simulink model "feedback_zd"  (R2022b)
settings: Solver=FixedStepAuto  StartTime=0.0  StopTime=15  FixedStep=0.001  RelTol=10-6
model workspace (MAT data in the model file):
  kd1 = Simulink.Parameter
  kd1.Value = 2
  kd1.DataType = 'auto'
  kd1.Complexity = 'real'
  kd1.Dimensions = [1 1]
  kd2 = Simulink.Parameter
  kd2.Value = 2
  kd2.DataType = 'auto'
  kd2.Complexity = 'real'
  kd2.Dimensions = [1 1]
  kp1 = Simulink.Parameter
  kp1.Value = 2
  kp1.DataType = 'auto'
  kp1.Complexity = 'real'
  kp1.Dimensions = [1 1]
  kp2 = Simulink.Parameter
  kp2.Value = 2
  kp2.DataType = 'auto'
  kp2.Complexity = 'real'
  kp2.Dimensions = [1 1]
values from neighbouring files (symbols this model uses):
  k_d1 = 50    [gains.m]
  k_d2 = 50    [gains.m]
  k_p1 = 30    [gains.m]
  k_p2 = 30    [gains.m]
undefined symbols (not defined in the file or in its folder): obstacle_x, obstacle_y, overtake_data, overtake_time
libraries: robotmobilelib x4
settings Model: Creator=thoma  LastModifiedBy=thoma
settings DebuggingCC: AlgebraicLoopMsg=none  UnderSpecifiedDimensionMsg=warning

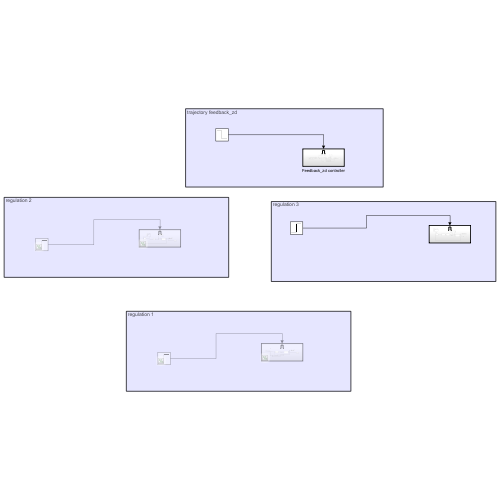
[thumbnail: Simulink's stored preview of the top-level diagram]
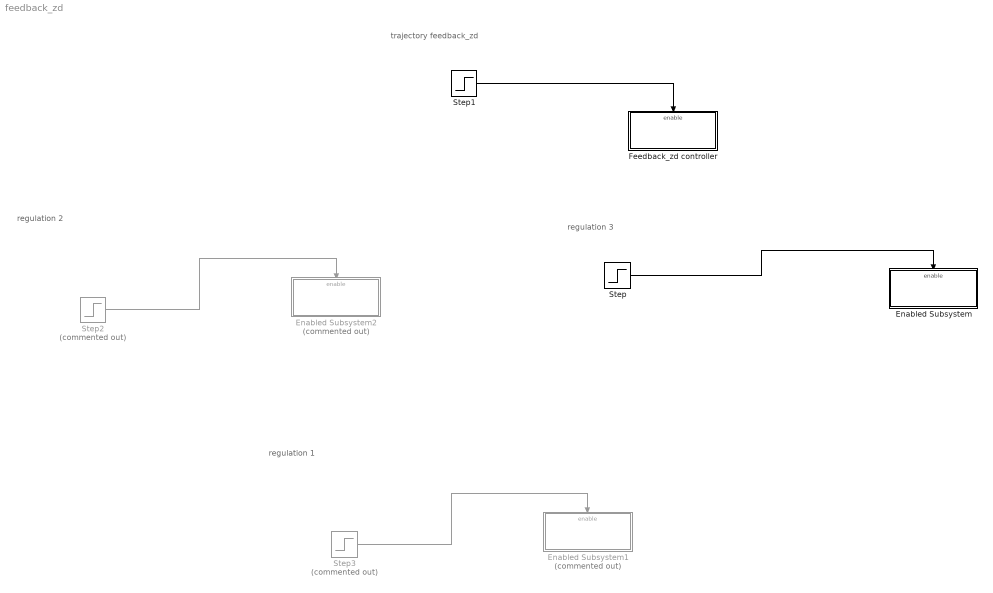
== system feedback_zd ==
  note: regulation 1
  note: regulation 3
  note: regulation 2
  note: trajectory feedback_zd
  Enabled Subsystem : Subsystem  TreatAsAtomicUnit=on
  Enabled Subsystem1 : Subsystem  Commented=on  TreatAsAtomicUnit=on
  Enabled Subsystem2 : Subsystem  Commented=on  TreatAsAtomicUnit=on
  Feedback_zd controller : Subsystem  TreatAsAtomicUnit=on
  Step : Step  Time=10  SampleTime=0
  Step1 : Step  Time=10  Before=1  After=0  SampleTime=0
  Step2 : Step  Commented=on  Time=10  SampleTime=0
  Step3 : Step  Commented=on  Time=10  SampleTime=0
  wires:
  Step3/1 -> Enabled Subsystem1/Enable
  Step1/1 -> Feedback_zd controller/Enable
  Step2/1 -> Enabled Subsystem2/Enable
  Step/1 -> Enabled Subsystem/Enable

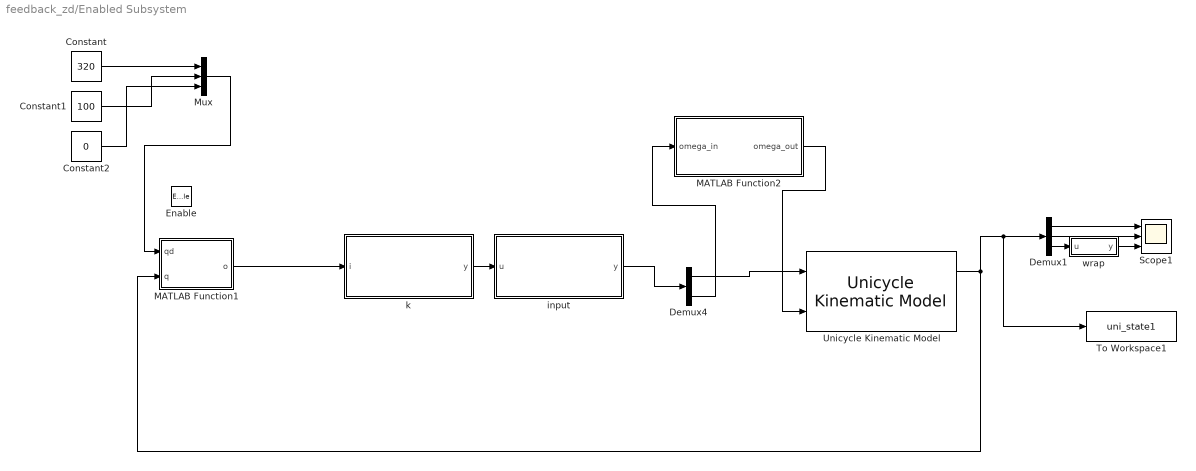
== system feedback_zd/Enabled Subsystem ==
  Enable : EnablePort
  Constant : Constant  Value=320
  Constant1 : Constant  Value=100
  Constant2 : Constant  Value=0
  Demux1 : Demux  Outputs=3
  Demux4 : Demux  Outputs=2
  MATLAB Function1 : MATLAB Function  TreatAsAtomicUnit=on
  MATLAB Function2 : MATLAB Function  TreatAsAtomicUnit=on
  Mux : Mux  Inputs=3
  Scope1 : Scope  NumInputPorts=3
  To Workspace1 : ToWorkspace  VariableName=uni_state1  SaveFormat=Structure With Time  SampleTime=0.001
  Unicycle Kinematic Model : robotmobilelib/Unicycle Kinematic Model  VehicleInputs=Vehicle Speed & Heading Angular Velocity  WheelRadius=2  WheelSpeedRange=[-Inf Inf]  InitialState=[125,60,0]  SimulateUsing=Interpreted execution
  input : MATLAB Function  TreatAsAtomicUnit=on
  k : MATLAB Function  TreatAsAtomicUnit=on
  wrap : MATLAB Function  TreatAsAtomicUnit=on
  wires:
  Constant/1 -> Mux/1
  Constant1/1 -> Mux/2
  Constant2/1 -> Mux/3
  Demux1/2 -> Scope1/2
  wrap/1(y) -> Scope1/3
  Unicycle Kinematic Model/1 -> To Workspace1/1, Demux1/1, MATLAB Function1/2(q)
  input/1(y) -> Demux4/1
  Demux1/3 -> wrap/1(u)
  k/1(y) -> input/1(u)
  Demux1/1 -> Scope1/1
  MATLAB Function1/1(o) -> k/1(i)
  Demux4/1 -> Unicycle Kinematic Model/1
  Mux/1 -> MATLAB Function1/1(qd)
  Demux4/2 -> MATLAB Function2/1(omega_in)
  MATLAB Function2/1(omega_out) -> Unicycle Kinematic Model/2

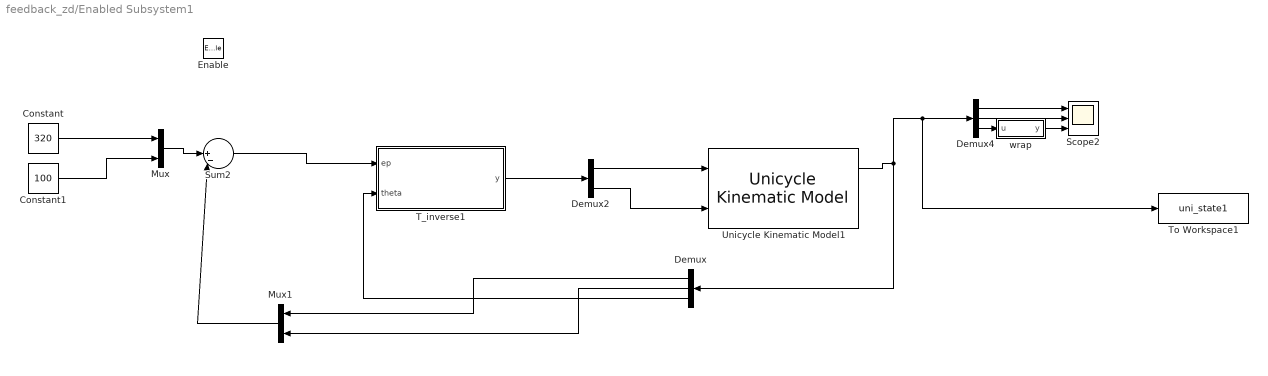
== system feedback_zd/Enabled Subsystem1 ==
  Enable : EnablePort
  Constant : Constant  Value=320
  Constant1 : Constant  Value=100
  Demux : Demux  Outputs=3
  Demux2 : Demux  Outputs=2
  Demux4 : Demux  Outputs=3
  Mux : Mux  Inputs=2
  Mux1 : Mux  Inputs=2
  Scope2 : Scope  NumInputPorts=3
  Sum2 : Sum  Inputs=||+-|
  T_inverse1 : MATLAB Function  TreatAsAtomicUnit=on
  To Workspace1 : ToWorkspace  VariableName=uni_state1  SaveFormat=Structure With Time  SampleTime=0.001
  Unicycle Kinematic Model1 : robotmobilelib/Unicycle Kinematic Model  VehicleInputs=Vehicle Speed & Heading Angular Velocity  WheelRadius=2  WheelSpeedRange=[-Inf Inf]  InitialState=[125,60,0]  SimulateUsing=Interpreted execution
  wrap : MATLAB Function  TreatAsAtomicUnit=on
  wires:
  wrap/1(y) -> Scope2/3
  Demux4/1 -> Scope2/1
  Demux4/2 -> Scope2/2
  Demux4/3 -> wrap/1(u)
  Sum2/1 -> T_inverse1/1(ep)
  Demux/1 -> Mux1/1
  Demux2/2 -> Unicycle Kinematic Model1/2
  Mux1/1 -> Sum2/2
  Demux2/1 -> Unicycle Kinematic Model1/1
  Unicycle Kinematic Model1/1 -> To Workspace1/1, Demux4/1, Demux/1
  T_inverse1/1(y) -> Demux2/1
  Demux/2 -> Mux1/2
  Demux/3 -> T_inverse1/2(theta)
  Constant1/1 -> Mux/2
  Constant/1 -> Mux/1
  Mux/1 -> Sum2/1

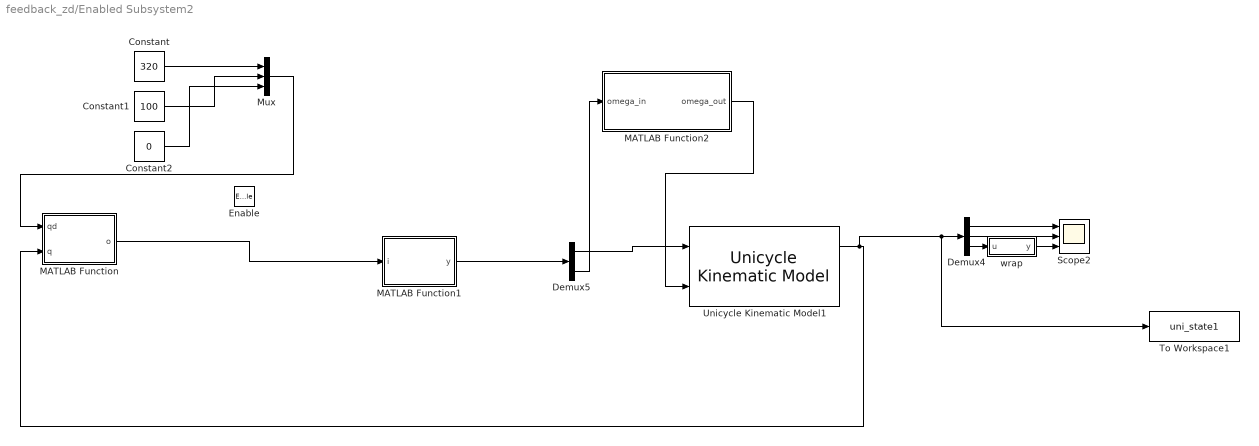
== system feedback_zd/Enabled Subsystem2 ==
  Enable : EnablePort
  Constant : Constant  Value=320
  Constant1 : Constant  Value=100
  Constant2 : Constant  Value=0
  Demux4 : Demux  Outputs=3
  Demux5 : Demux  Outputs=2
  MATLAB Function : MATLAB Function  TreatAsAtomicUnit=on
  MATLAB Function1 : MATLAB Function  TreatAsAtomicUnit=on
  MATLAB Function2 : MATLAB Function  TreatAsAtomicUnit=on
  Mux : Mux  Inputs=3
  Scope2 : Scope  NumInputPorts=3
  To Workspace1 : ToWorkspace  VariableName=uni_state1  SaveFormat=Structure With Time  SampleTime=0.001
  Unicycle Kinematic Model1 : robotmobilelib/Unicycle Kinematic Model  VehicleInputs=Vehicle Speed & Heading Angular Velocity  WheelRadius=2  WheelSpeedRange=[-Inf Inf]  InitialState=[125,60,0]  SimulateUsing=Interpreted execution
  wrap : MATLAB Function  TreatAsAtomicUnit=on
  wires:
  Demux5/1 -> Unicycle Kinematic Model1/1
  wrap/1(y) -> Scope2/3
  MATLAB Function/1(o) -> MATLAB Function1/1(i)
  MATLAB Function1/1(y) -> Demux5/1
  Demux4/1 -> Scope2/1
  Demux4/2 -> Scope2/2
  Demux4/3 -> wrap/1(u)
  Unicycle Kinematic Model1/1 -> To Workspace1/1, Demux4/1, MATLAB Function/2(q)
  Constant/1 -> Mux/1
  Constant1/1 -> Mux/2
  Constant2/1 -> Mux/3
  Mux/1 -> MATLAB Function/1(qd)
  Demux5/2 -> MATLAB Function2/1(omega_in)
  MATLAB Function2/1(omega_out) -> Unicycle Kinematic Model1/2

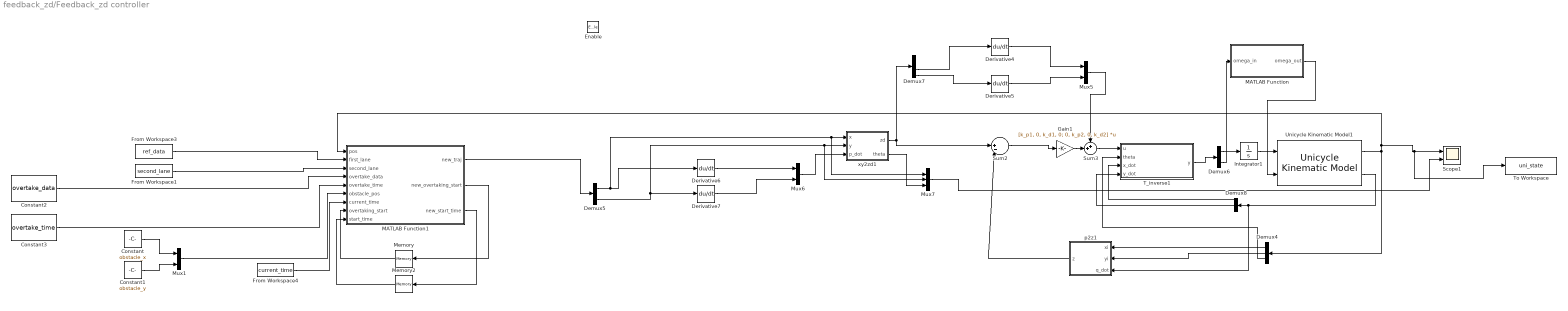
== system feedback_zd/Feedback_zd controller ==
  Enable : EnablePort
  Constant : Constant  Value=obstacle_x
  Constant1 : Constant  Value=obstacle_y
  Constant2 : Constant  Value=overtake_data
  Constant3 : Constant  Value=overtake_time
  Demux4 : Demux  Outputs=3
  Demux5 : Demux  Outputs=2
  Demux6 : Demux  Outputs=2
  Demux7 : Demux
  Demux8 : Demux  Outputs=3
  Derivative{4..7} (4 alike) : Derivative
  From Workspace1 : FromWorkspace  VariableName=second_lane
  From Workspace3 : FromWorkspace  VariableName=ref_data
  From Workspace4 : FromWorkspace  VariableName=current_time
  Gain1 : Gain  Gain=[k_p1, 0, k_d1, 0; 0, k_p2, 0, k_d2]  Multiplication=Matrix(K*u)
  Integrator1 : Integrator
  MATLAB Function : MATLAB Function  TreatAsAtomicUnit=on
  MATLAB Function1 : MATLAB Function  TreatAsAtomicUnit=on
  Memory : Memory
  Memory2 : Memory
  Mux1 : Mux  Inputs=2
  Mux5 : Mux  Inputs=2
  Mux6 : Mux  Inputs=2
  Mux7 : Mux  Inputs=3
  Scope1 : Scope  NumInputPorts=2
  Sum2 : Sum  Inputs=||+-|
  Sum3 : Sum  Inputs=++|
  T_inverse1 : MATLAB Function  TreatAsAtomicUnit=on
  To Workspace : ToWorkspace  VariableName=uni_state  SaveFormat=Structure With Time  SampleTime=0.01
  Unicycle Kinematic Model1 : robotmobilelib/Unicycle Kinematic Model  VehicleInputs=Vehicle Speed & Heading Angular Velocity  WheelRadius=2  WheelSpeedRange=[-Inf Inf]  InitialState=[125; 60; 0]  SimulateUsing=Interpreted execution
  p2z1 : MATLAB Function  TreatAsAtomicUnit=on
  xy2zd1 : MATLAB Function  TreatAsAtomicUnit=on
  wires:
  Demux4/1 -> p2z1/1(xi)
  Sum3/1 -> T_inverse1/1(u)
  Mux5/1 -> Sum3/1
  xy2zd1/1(zd) -> Demux7/1, Sum2/1
  p2z1/1(z) -> Sum2/2
  Demux4/3 -> T_inverse1/2(theta)
  Demux5/2 -> Mux7/2, xy2zd1/2(y), Derivative7/1
  Derivative6/1 -> Mux6/1
  Derivative7/1 -> Mux6/2
  Demux6/1 -> Integrator1/1
  T_inverse1/1(y) -> Demux6/1
  Demux8/2 -> T_inverse1/4(y_dot)
  MATLAB Function1/1(new_traj) -> Demux5/1
  Sum2/1 -> Gain1/1
  Demux7/4 -> Derivative5/1
  Unicycle Kinematic Model1/2 -> p2z1/3(q_dot), Demux8/1
  Demux5/1 -> Mux7/1, xy2zd1/1(x), Derivative6/1
  Integrator1/1 -> Unicycle Kinematic Model1/1
  Demux7/3 -> Derivative4/1
  Derivative5/1 -> Mux5/2
  Mux7/1 -> Scope1/2
  Demux6/2 -> MATLAB Function/1(omega_in)
  Gain1/1 -> Sum3/2
  Unicycle Kinematic Model1/1 -> MATLAB Function1/1(pos), To Workspace/1, Scope1/1, Demux4/1
  MATLAB Function/1(omega_out) -> Unicycle Kinematic Model1/2
  Derivative4/1 -> Mux5/1
  Demux4/2 -> p2z1/2(yi)
  Mux6/1 -> xy2zd1/3(p_dot)
  Demux8/1 -> T_inverse1/3(x_dot)
  Memory2/1 -> MATLAB Function1/9(start_time)
  Constant3/1 -> MATLAB Function1/5(overtake_time)
  Constant2/1 -> MATLAB Function1/4(overtake_data)
  From Workspace1/1 -> MATLAB Function1/3(second_lane)
  Mux1/1 -> MATLAB Function1/6(obstacle_pos)
  From Workspace4/1 -> MATLAB Function1/7(current_time)
  Constant1/1 -> Mux1/2
  Memory/1 -> MATLAB Function1/8(overtaking_start)
  From Workspace3/1 -> MATLAB Function1/2(first_lane)
  MATLAB Function1/2(new_overtaking_start) -> Memory/1
  Constant/1 -> Mux1/1
  MATLAB Function1/3(new_start_time) -> Memory2/1
  xy2zd1/2(theta) -> Mux7/3

== matlab function feedback_zd/Enabled Subsystem1/wrap ==
  data: u input; y output
function y = fcn(u)

y =mod(u+pi,2*pi)-pi;

== matlab function feedback_zd/Enabled Subsystem1/T_inverse1 ==
  data: ep input; y output; theta input
function y = fcn(ep,theta)
theta=mod(theta+pi,2*pi)-pi;
kv=40;
kw=50;
v=kv*(ep(1)*cos(theta)+ep(2)*sin(theta));
w=kw*(atan2(-ep(2),-ep(1))+pi-theta);
y = [v;w];

== matlab function feedback_zd/Feedback_zd controller/MATLAB Function ==
  data: omega_in input; omega_out output
function omega_out = check_omega(omega_in)
    % Check if omega (angular velocity) is finite
    if ~isfinite(omega_in)
        omega_out = 0;  % Set omega to a default value, e.g., 0 if it is NaN or Inf
    else
        omega_out = omega_in;  % Otherwise, pass the input value
    end
end

== matlab function feedback_zd/Feedback_zd controller/T_inverse1 ==
  data: u input; y output; theta input; x_dot input; y_dot input
function y = fcn(u,theta,x_dot,y_dot)
v=sqrt(x_dot^2+y_dot^2);
theta=mod(theta+pi,2*pi)-pi;
T_inverse=[cos(theta),sin(theta);-sin(theta)/v,cos(theta)/v];
vet=T_inverse*u;
y = vet;

== matlab function feedback_zd/Feedback_zd controller/p2z1 ==
  data: xi input; yi input; z output; q_dot input
function z = fcn(xi,yi, q_dot)
x_dot = q_dot(1);
y_dot = q_dot(2);
z = [xi; yi; x_dot; y_dot];  % z is a 4x1 vecto

== matlab function feedback_zd/Feedback_zd controller/xy2zd1 ==
  data: x input; y input; zd output; p_dot input; theta output
function [zd, theta]= fcn(x,y,p_dot)
v_x = p_dot(1);
if abs(v_x) <= 1e-4
    v_x = sign(v_x)*1e-4;
end
v_y = p_dot(2);
v = sqrt(v_x^2 + v_y^2);
theta = atan2(v_y, v_x);
theta=mod(theta+pi,2*pi)-pi;
z3=v*cos(theta);
z4=v*sin(theta);
zd=[x;y;z3;z4];

== matlab function feedback_zd/Enabled Subsystem/MATLAB Function1 ==
  data: qd input; o output; q input
function o = fcn(qd,q)
xi=q(1);
yi=q(2);
thetai=q(3);
x=-(qd(1)-xi);
y=-(qd(2)-yi);
theta=-(qd(3)-thetai);
theta=mod(theta+pi,2*pi)-pi;
rho=sqrt(x^2+y^2);
gamma=atan2(y,x)+pi-theta;
delta=gamma+theta;
delta=mod(delta+pi,2*pi)-pi;
gamma=mod(gamma+pi,2*pi)-pi;
o = [rho;gamma;delta];

== matlab function feedback_zd/Enabled Subsystem/MATLAB Function2 ==
  data: omega_in input; omega_out output
function omega_out = check_omega(omega_in)
    % Check if omega (angular velocity) is finite
    if ~isfinite(omega_in)
        omega_out = 0;  % Set omega to a default value, e.g., 0 if it is NaN or Inf
    else
        omega_out = omega_in;  % Otherwise, pass the input value
    end
end

== matlab function feedback_zd/Feedback_zd controller/MATLAB Function1 ==
  data: pos input; first_lane input; new_traj output; second_lane input; overtake_data input; overtake_time input; obstacle_pos input size=[2]; current_time input; overtaking_start input; new_overtaking_start output; new_start_time output; start_time input
function [new_traj, new_overtaking_start, new_start_time]  = fcn(pos,first_lane, second_lane, overtake_data, overtake_time, obstacle_pos, current_time, overtaking_start, start_time)
detection_margin_x = 85; % Detection range in x-direction
detection_margin_y = 55; % Detection range in y-direction
early_detection_distance = 60; % Distance ahead of obstacle to start overtaking
% Check if obstacle is within detection range and ahead of the obstacle   
if ~overtaking_start   
    if (abs(pos(1) - obstacle_pos(1)) < detection_margin_x && abs(pos(2) - obstacle_pos(2)) < detection_margin_y) && pos(1) < obstacle_pos(1) + early_detection_distance
        new_overtaking_start = 1;
        new_start_time = current_time;
    else
        new_overtaking_start = overtaking_start;
        new_start_time = start_time;
    end
    idx = 1;
else
    idx = find(abs(overtake_time - (current_time - start_time)) <= 1e-3, 1);
    if ~isempty(idx)
        new_overtaking_start = overtaking_start;
    else
        new_overtaking_start = 0;
        idx = 1;
    end
    new_start_time = start_time;
end
new_traj = first_lane + (second_lane-first_lane)*overtake_data(idx);

== matlab function feedback_zd/Enabled Subsystem/input ==
  data: u input; y output
function y = fcn(u)
v=u(2)*u(1);
w=u(3);
y = [v;w];

== matlab function feedback_zd/Enabled Subsystem2/MATLAB Function ==
  data: qd input; o output; q input
function o = fcn(qd,q)
xi=q(1);
yi=q(2);
thetai=q(3);
x=-(qd(1)-xi);
y=-(qd(2)-yi);
theta=-(qd(3)-thetai);
rho=sqrt(x^2+y^2);
gamma=atan2(y,x)+pi-theta;
delta=gamma+theta;
delta=mod(delta+pi,2*pi)-pi;
gamma=mod(gamma+pi,2*pi)-pi;
o = [rho;gamma;delta];

== matlab function feedback_zd/Enabled Subsystem2/MATLAB Function1 ==
  data: i input; y output
function y = fcn(i)
k1=20;
k2=30;
k3=4;
rho=i(1);
gamma=i(2);
delta=i(3);
v=k1*rho*cos(gamma);
w=k2*gamma+(k1* ((sin(gamma)*cos(gamma))/gamma) * (gamma+k3*delta));
y = [v;w];

== matlab function feedback_zd/Enabled Subsystem2/MATLAB Function2 ==
  data: omega_in input; omega_out output
function omega_out = check_omega(omega_in)
    % Check if omega (angular velocity) is finite
    if ~isfinite(omega_in)
        omega_out = 0;  % Set omega to a default value, e.g., 0 if it is NaN or Inf
    else
        omega_out = omega_in;  % Otherwise, pass the input value
    end
end

== matlab function feedback_zd/Enabled Subsystem2/wrap ==
  data: u input; y output
function y = fcn(u)

y =mod(u+pi,2*pi)-pi;

== matlab function feedback_zd/Enabled Subsystem/k ==
  data: i input; y output
function y = fcn(i)
k1=20;
k2=100;
k3=20;
rho=i(1);
gamma=i(2);
delta=i(3);
u=k1*cos(gamma);
w=k2*gamma+(k1* ((sin(gamma)*cos(gamma))/gamma) * (gamma+k3*delta));
y = [rho;u;w];

== matlab function feedback_zd/Enabled Subsystem/wrap ==
  data: u input; y output
function y = fcn(u)

y =mod(u+pi,2*pi)-pi;
